simulink model "cieplo_budynek_otoczenie"  (R2020b)
settings: Solver=VariableStepAuto  StartTime=0.0  StopTime=48  RelTol=1e-3
settings Model: Creator=matis  LastModifiedBy=matis

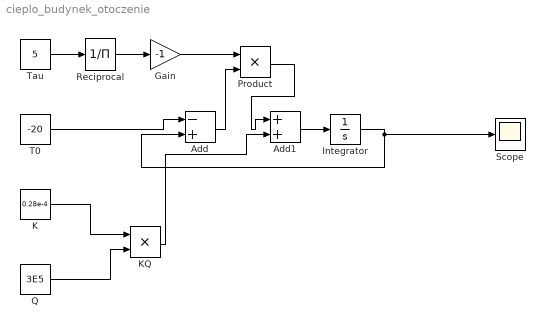
== system cieplo_budynek_otoczenie ==
  Add : Sum  Inputs=-+
  Add1 : Sum
  Gain : Gain  Gain=-1
  Integrator : Integrator  InitialCondition=15
  K : Constant  Value=0.28e-4
  KQ : Product
  Product : Product
  Q : Constant  Value=3E5
  Reciprocal : Product  Inputs=/
  Scope : Scope
  T0 : Constant  Value=-20
  Tau : Constant  Value=5
  wires:
  K/1 -> KQ/1
  Q/1 -> KQ/2
  Tau/1 -> Reciprocal/1
  Reciprocal/1 -> Gain/1
  T0/1 -> Add/1
  Integrator/1 -> Add/2, Scope/1
  Gain/1 -> Product/1
  Add/1 -> Product/2
  KQ/1 -> Add1/2
  Product/1 -> Add1/1
  Add1/1 -> Integrator/1
